simulink model "Observer_Exp1"  (R2019a)
settings: Solver=VariableStepAuto  StartTime=0.0  StopTime=2  MaxStep=.001  RelTol=1e-3
settings Model: Creator=aaami  LastModifiedBy=aaami

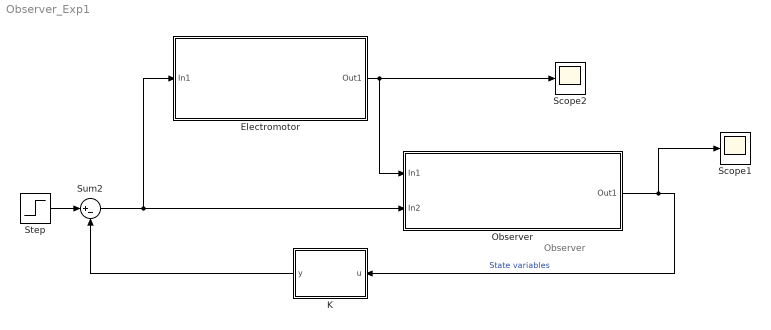
== system Observer_Exp1 ==
  note: Observer
  Electromotor : Subsystem
  K : MATLAB Function  TreatAsAtomicUnit=on
  Observer : Subsystem
  Scope1 : Scope
  Scope2 : Scope
  Step : Step  Time=0  SampleTime=0
  Sum2 : Sum  Inputs=|+-
  wires:
  Step/1 -> Sum2/1
  Sum2/1 -> Observer/2(In2), Electromotor/1(In1)
  K/1(y) -> Sum2/2
  Electromotor/1(Out1) -> Observer/1(In1), Scope2/1
  Observer/1(Out1) -> Scope1/1, K/1(u)  "State variables"

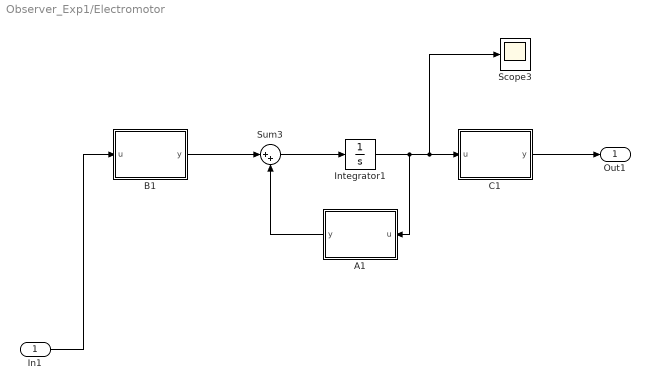
== system Observer_Exp1/Electromotor ==
  In1 : Inport
  A1 : MATLAB Function  TreatAsAtomicUnit=on
  B1 : MATLAB Function  TreatAsAtomicUnit=on
  C1 : MATLAB Function  TreatAsAtomicUnit=on
  Integrator1 : Integrator  InitialCondition=[0;0]
  Scope3 : Scope
  Sum3 : Sum  Inputs=|++
  Out1 : Outport
  wires:
  In1/1 -> B1/1(u)
  Integrator1/1 -> A1/1(u), Scope3/1, C1/1(u)
  Sum3/1 -> Integrator1/1
  A1/1(y) -> Sum3/2
  C1/1(y) -> Out1/1
  B1/1(y) -> Sum3/1

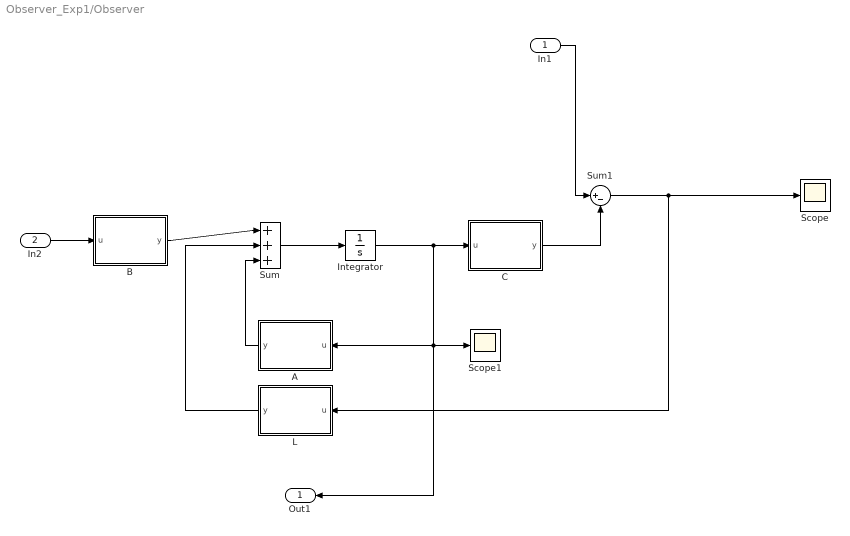
== system Observer_Exp1/Observer ==
  In1 : Inport
  In2 : Inport  Port=2
  A : MATLAB Function  TreatAsAtomicUnit=on
  B : MATLAB Function  TreatAsAtomicUnit=on
  C : MATLAB Function  TreatAsAtomicUnit=on
  Integrator : Integrator  InitialCondition=[0.01;0]
  L : MATLAB Function  TreatAsAtomicUnit=on
  Scope : Scope
  Scope1 : Scope
  Sum : Sum  Inputs=|+++
  Sum1 : Sum  Inputs=|+-
  Out1 : Outport
  wires:
  Integrator/1 -> Out1/1, Scope1/1, A/1(u), C/1(u)
  Sum1/1 -> L/1(u), Scope/1
  A/1(y) -> Sum/3
  Sum/1 -> Integrator/1
  B/1(y) -> Sum/1
  C/1(y) -> Sum1/2
  L/1(y) -> Sum/2
  In2/1 -> B/1(u)
  In1/1 -> Sum1/1

== matlab function Observer_Exp1/Observer/A ==
  data: u input; y output
function y = fcn(u)
A=[ -4 1
    0 0];
y = A*u;

== matlab function Observer_Exp1/Observer/C ==
  data: u input; y output
function y = fcn(u)
C=[1 0 ];
y = C*u;

== matlab function Observer_Exp1/Observer/L ==
  data: u input; y output
function y = fcn(u)
L=[156;6519];
y = L*u;

== matlab function Observer_Exp1/Observer/B ==
  data: u input; y output
function y = fcn(u)
B=[0;1];
y = B*u;

== matlab function Observer_Exp1/Electromotor/B1 ==
  data: u input; y output
function y = fcn(u)
B=[0;1];
y = B*u;

== matlab function Observer_Exp1/Electromotor/C1 ==
  data: u input; y output
function y = fcn(u)
C=[1 0 ];
y = C*u;

== matlab function Observer_Exp1/Electromotor/A1 ==
  data: u input; y output
function y = fcn(u)
A=[ -4 1
    0 0];
y = A*u;

== matlab function Observer_Exp1/K ==
  data: u input; y output
function y = fcn(u)
K=[135 12];
y = K*u;
